simulink model "SFS0"  (R2022b)
settings: Solver=FixedStepAuto  StartTime=0.0  StopTime=10.0  FixedStep=0.20000000000000001  RelTol=1e-3
undefined symbols (not defined in the file): ACCELERATION_MAX, covA, covarience_matrix_IC, covG, covM, covP, covV, fusion_t, gps_ratio, location_lla_IC, MAG_MAX, noise_state, POS_MAX, state_IC, VELOCITY_MAX, YAW_MAX
settings Model: DVExtractedSubsystem=SFS  Creator=Inver  LastModifiedBy=Inver
settings DebuggingCC: SignalRangeChecking=warning  FrameProcessingCompatibilityMsg=none
settings RTWCC: TLCOptions=-aAlwaysIncludeCustomSrc=1

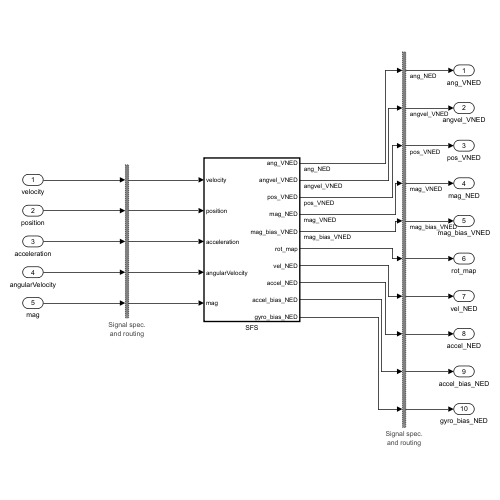
[thumbnail: Simulink's stored preview of the top-level diagram]
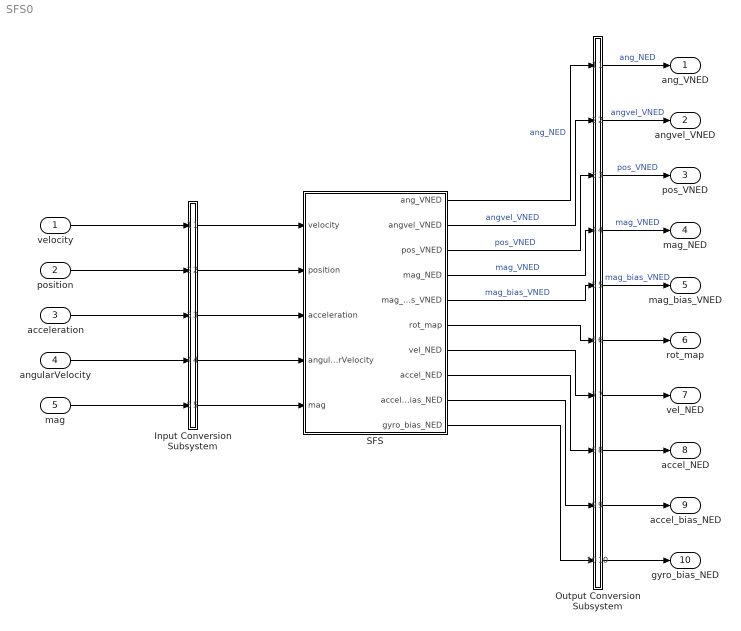
== system SFS0 ==
  velocity : Inport  OutMin=-30  OutMax=30  OutDataTypeStr=double  PortDimensions=[3, 1]  SampleTime=0.2  Interpolate=off
  position : Inport  Port=2  OutMin=-300  OutMax=300  OutDataTypeStr=double  PortDimensions=[3, 1]  SampleTime=0.2  Interpolate=off
  acceleration : Inport  Port=3  OutMin=-30  OutMax=30  OutDataTypeStr=double  PortDimensions=[3, 1]  SampleTime=0.2  Interpolate=off
  angularVelocity : Inport  Port=4  OutMin=-2.5  OutMax=2.5  OutDataTypeStr=double  PortDimensions=[3, 1]  SampleTime=0.2  Interpolate=off
  mag : Inport  Port=5  OutMin=-200  OutMax=200  OutDataTypeStr=double  PortDimensions=[3, 1]  SampleTime=0.2  Interpolate=off
  Input Conversion Subsystem : Subsystem  Tag=__SLT_ICS__  Description=|
      | Signal spec.
      | and routing
      settings: AttributesFormatString=%<Description>
  Output Conversion Subsystem : Subsystem  Tag=__SLT_OCS__  Description=|
      | Signal spec.
      | and routing
      settings: AttributesFormatString=%<Description>
  SFS : Subsystem  TreatAsAtomicUnit=on
  ang_VNED : Outport
  angvel_VNED : Outport  Port=2
  pos_VNED : Outport  Port=3
  mag_NED : Outport  Port=4
  mag_bias_VNED : Outport  Port=5
  rot_map : Outport  Port=6
  vel_NED : Outport  Port=7
  accel_NED : Outport  Port=8
  accel_bias_NED : Outport  Port=9
  gyro_bias_NED : Outport  Port=10
  wires:
  velocity/1 -> Input Conversion Subsystem/1(Inport_1)
  position/1 -> Input Conversion Subsystem/2(Inport_2)
  acceleration/1 -> Input Conversion Subsystem/3(Inport_3)
  angularVelocity/1 -> Input Conversion Subsystem/4(Inport_4)
  mag/1 -> Input Conversion Subsystem/5(Inport_5)
  Output Conversion Subsystem/1(Outport_1) -> ang_VNED/1  "ang_NED"
  Output Conversion Subsystem/2(Outport_2) -> angvel_VNED/1  "angvel_VNED"
  Output Conversion Subsystem/3(Outport_3) -> pos_VNED/1  "pos_VNED"
  Output Conversion Subsystem/4(Outport_4) -> mag_NED/1  "mag_VNED"
  Output Conversion Subsystem/5(Outport_5) -> mag_bias_VNED/1  "mag_bias_VNED"
  Output Conversion Subsystem/6(Outport_6) -> rot_map/1
  Output Conversion Subsystem/7(Outport_7) -> vel_NED/1
  Output Conversion Subsystem/8(Outport_8) -> accel_NED/1
  Output Conversion Subsystem/9(Outport_9) -> accel_bias_NED/1
  Output Conversion Subsystem/10(Outport_10) -> gyro_bias_NED/1
  Input Conversion Subsystem/1(Outport_1) -> SFS/1(velocity)
  Input Conversion Subsystem/2(Outport_2) -> SFS/2(position)
  Input Conversion Subsystem/3(Outport_3) -> SFS/3(acceleration)
  Input Conversion Subsystem/4(Outport_4) -> SFS/4(angularVelocity)
  Input Conversion Subsystem/5(Outport_5) -> SFS/5(mag)
  SFS/1(ang_VNED) -> Output Conversion Subsystem/1(Inport_1)  "ang_NED"
  SFS/2(angvel_VNED) -> Output Conversion Subsystem/2(Inport_2)  "angvel_VNED"
  SFS/3(pos_VNED) -> Output Conversion Subsystem/3(Inport_3)  "pos_VNED"
  SFS/4(mag_NED) -> Output Conversion Subsystem/4(Inport_4)  "mag_VNED"
  SFS/5(mag_bias_VNED) -> Output Conversion Subsystem/5(Inport_5)  "mag_bias_VNED"
  SFS/6(rot_map) -> Output Conversion Subsystem/6(Inport_6)
  SFS/7(vel_NED) -> Output Conversion Subsystem/7(Inport_7)
  SFS/8(accel_NED) -> Output Conversion Subsystem/8(Inport_8)
  SFS/9(accel_bias_NED) -> Output Conversion Subsystem/9(Inport_9)
  SFS/10(gyro_bias_NED) -> Output Conversion Subsystem/10(Inport_10)

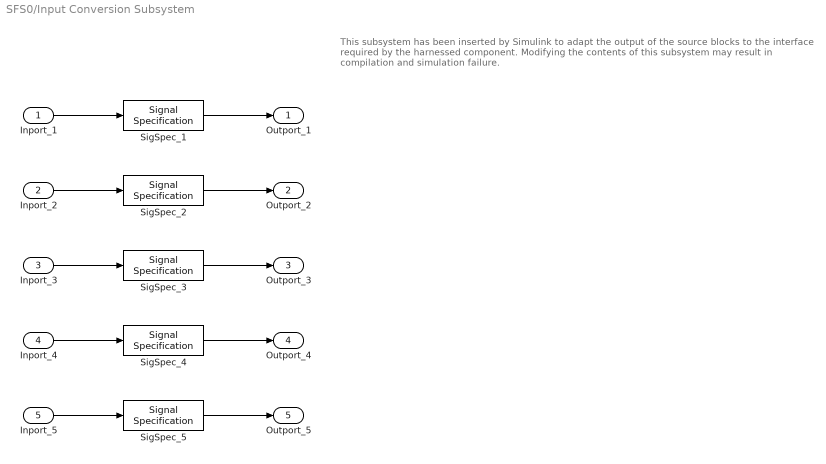
== system SFS0/Input Conversion Subsystem ==
  note: This subsystem has been inserted by Simulink to adapt the output of the source blocks to the interface required by the harnessed component.
      |  Modifying the contents of this subsystem may result in compilation and simulation failure.
  Inport_1 : Inport
  Inport_2 : Inport  Port=2
  Inport_3 : Inport  Port=3
  Inport_4 : Inport  Port=4
  Inport_5 : Inport  Port=5
  SigSpec_{1..5} (5 alike) : SignalSpecification  OutDataTypeStr=double  Dimensions=[3, 1]  SampleTime=0.2
  Outport_1 : Outport
  Outport_2 : Outport  Port=2
  Outport_3 : Outport  Port=3
  Outport_4 : Outport  Port=4
  Outport_5 : Outport  Port=5
  wires:
  SigSpec_1/1 -> Outport_1/1
  Inport_1/1 -> SigSpec_1/1
  SigSpec_2/1 -> Outport_2/1
  Inport_2/1 -> SigSpec_2/1
  SigSpec_3/1 -> Outport_3/1
  Inport_3/1 -> SigSpec_3/1
  SigSpec_4/1 -> Outport_4/1
  Inport_4/1 -> SigSpec_4/1
  SigSpec_5/1 -> Outport_5/1
  Inport_5/1 -> SigSpec_5/1

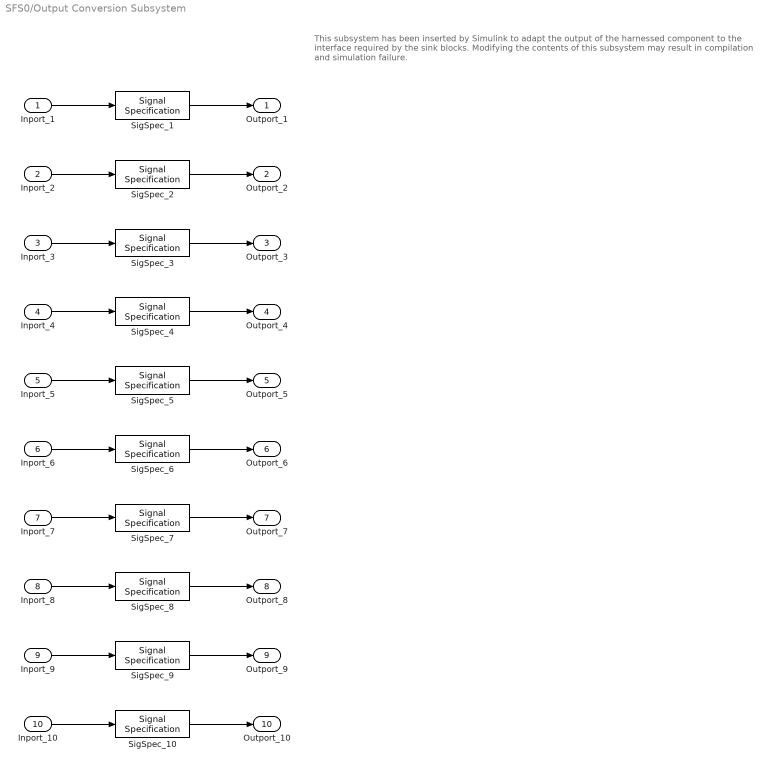
== system SFS0/Output Conversion Subsystem ==
  note: This subsystem has been inserted by Simulink to adapt the output of the harnessed component to the interface required by the sink blocks.
      |  Modifying the contents of this subsystem may result in compilation and simulation failure.
  Inport_1 : Inport
  Inport_2 : Inport  Port=2
  Inport_3 : Inport  Port=3
  Inport_4 : Inport  Port=4
  Inport_5 : Inport  Port=5
  Inport_6 : Inport  Port=6
  Inport_7 : Inport  Port=7
  Inport_8 : Inport  Port=8
  Inport_9 : Inport  Port=9
  Inport_10 : Inport  Port=10
  SigSpec_1 : SignalSpecification  OutDataTypeStr=double  Dimensions=[4, 1]  SampleTime=0.2
  SigSpec_{2..5,7..10} (8 alike) : SignalSpecification  OutDataTypeStr=double  Dimensions=[3, 1]  SampleTime=0.2
  SigSpec_6 : SignalSpecification  OutDataTypeStr=double  Dimensions=[3, 3]  SampleTime=0.2
  Outport_1 : Outport
  Outport_2 : Outport  Port=2
  Outport_3 : Outport  Port=3
  Outport_4 : Outport  Port=4
  Outport_5 : Outport  Port=5
  Outport_6 : Outport  Port=6
  Outport_7 : Outport  Port=7
  Outport_8 : Outport  Port=8
  Outport_9 : Outport  Port=9
  Outport_10 : Outport  Port=10
  wires:
  Inport_1/1 -> SigSpec_1/1
  SigSpec_1/1 -> Outport_1/1
  Inport_2/1 -> SigSpec_2/1
  SigSpec_2/1 -> Outport_2/1
  Inport_3/1 -> SigSpec_3/1
  SigSpec_3/1 -> Outport_3/1
  Inport_4/1 -> SigSpec_4/1
  SigSpec_4/1 -> Outport_4/1
  Inport_5/1 -> SigSpec_5/1
  SigSpec_5/1 -> Outport_5/1
  Inport_6/1 -> SigSpec_6/1
  SigSpec_6/1 -> Outport_6/1
  Inport_7/1 -> SigSpec_7/1
  SigSpec_7/1 -> Outport_7/1
  Inport_8/1 -> SigSpec_8/1
  SigSpec_8/1 -> Outport_8/1
  Inport_9/1 -> SigSpec_9/1
  SigSpec_9/1 -> Outport_9/1
  Inport_10/1 -> SigSpec_10/1
  SigSpec_10/1 -> Outport_10/1

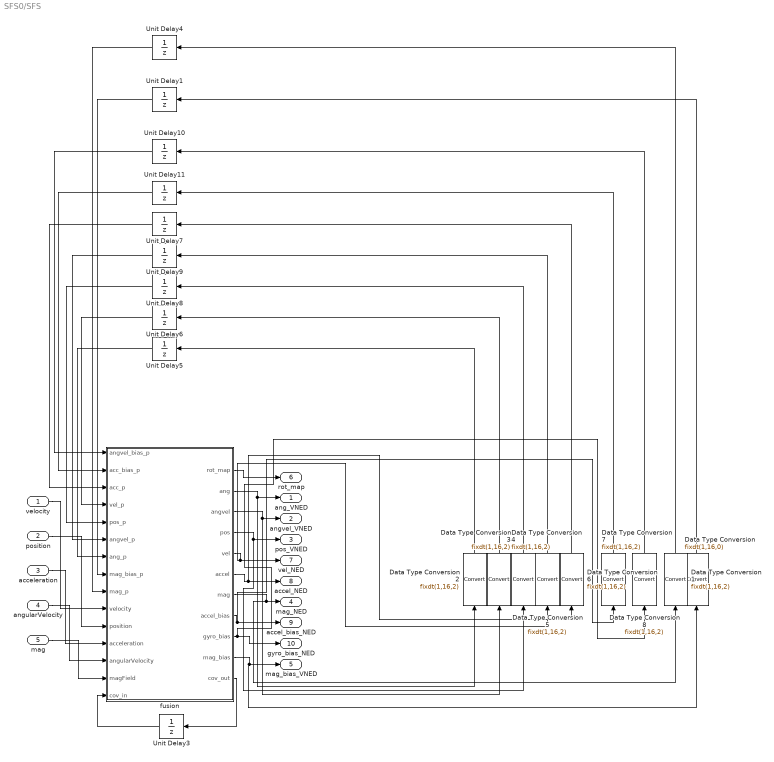
== system SFS0/SFS ==
  velocity : Inport  OutMin=-VELOCITY_MAX  OutMax=VELOCITY_MAX  OutDataTypeStr=double
  position : Inport  Port=2  OutMin=-POS_MAX  OutMax=POS_MAX  OutDataTypeStr=double
  acceleration : Inport  Port=3  OutMin=-ACCELERATION_MAX  OutMax=ACCELERATION_MAX  OutDataTypeStr=double  PortDimensions=[3 1]
  angularVelocity : Inport  Port=4  OutMin=-YAW_MAX  OutMax=YAW_MAX  OutDataTypeStr=double  PortDimensions=[3 1]
  mag : Inport  Port=5  OutMin=-MAG_MAX  OutMax=MAG_MAX  OutDataTypeStr=double  PortDimensions=[3 1]
  Data Type Conversion : DataTypeConversion  OutDataTypeStr=fixdt(1,16,0)  SaturateOnIntegerOverflow=off  RndMeth=Floor
  Data Type Conversion{1..8} (8 alike) : DataTypeConversion  OutDataTypeStr=fixdt(1,16,2)  SaturateOnIntegerOverflow=off  RndMeth=Floor
  Unit Delay1 : UnitDelay  InitialCondition=[0; 0; 0]  SampleTime=-1  HasFrameUpgradeWarning=on
  Unit Delay10 : UnitDelay  InitialCondition=state_IC(20:22)  SampleTime=-1  HasFrameUpgradeWarning=on
  Unit Delay11 : UnitDelay  InitialCondition=state_IC(17:19)  SampleTime=-1  HasFrameUpgradeWarning=on
  Unit Delay3 : UnitDelay  InitialCondition=covarience_matrix_IC  SampleTime=-1  HasFrameUpgradeWarning=on
  Unit Delay4 : UnitDelay  InitialCondition=mag_field_IC'  SampleTime=-1  HasFrameUpgradeWarning=on
  Unit Delay5 : UnitDelay  InitialCondition=state_IC(1:4)  SampleTime=-1  HasFrameUpgradeWarning=on
  Unit Delay6 : UnitDelay  InitialCondition=state_IC(5:7)  SampleTime=-1  HasFrameUpgradeWarning=on
  Unit Delay7 : UnitDelay  InitialCondition=state_IC(14:16)  SampleTime=-1  HasFrameUpgradeWarning=on
  Unit Delay8 : UnitDelay  InitialCondition=state_IC(8:10)  SampleTime=-1  HasFrameUpgradeWarning=on
  Unit Delay9 : UnitDelay  InitialCondition=state_IC(11:13)  SampleTime=-1  HasFrameUpgradeWarning=on
  fusion : MATLAB Function  TreatAsAtomicUnit=on
  ang_VNED : Outport  OutMin=-1  OutMax=1  OutDataTypeStr=double
  angvel_VNED : Outport  Port=2  OutMin=-YAW_MAX  OutMax=YAW_MAX  OutDataTypeStr=double
  pos_VNED : Outport  Port=3  OutMin=-POS_MAX  OutMax=POS_MAX  OutDataTypeStr=double
  mag_NED : Outport  Port=4  OutMin=-MAG_MAX  OutMax=MAG_MAX  OutDataTypeStr=double
  mag_bias_VNED : Outport  Port=5  OutMin=-MAG_MAX  OutMax=MAG_MAX  OutDataTypeStr=double
  rot_map : Outport  Port=6  OutMin=-1  OutMax=1  OutDataTypeStr=double
  vel_NED : Outport  Port=7  OutMin=-VELOCITY_MAX  OutMax=VELOCITY_MAX  OutDataTypeStr=double
  accel_NED : Outport  Port=8  OutMin=-ACCELERATION_MAX  OutMax=ACCELERATION_MAX  OutDataTypeStr=double
  accel_bias_NED : Outport  Port=9  OutMin=-ACCELERATION_MAX  OutMax=ACCELERATION_MAX  OutDataTypeStr=double
  gyro_bias_NED : Outport  Port=10  OutMin=-YAW_MAX  OutMax=YAW_MAX  OutDataTypeStr=double
  wires:
  Data Type Conversion8/1 -> Unit Delay10/1
  Data Type Conversion7/1 -> Unit Delay11/1
  Unit Delay10/1 -> fusion/1(angvel_bias_p)
  Unit Delay11/1 -> fusion/2(acc_bias_p)
  fusion/8(accel_bias) -> accel_bias_NED/1, Data Type Conversion7/1
  Unit Delay5/1 -> fusion/7(ang_p)
  Unit Delay9/1 -> fusion/6(angvel_p)
  Unit Delay8/1 -> fusion/5(pos_p)
  Unit Delay6/1 -> fusion/4(vel_p)
  Unit Delay7/1 -> fusion/3(acc_p)
  Data Type Conversion6/1 -> Unit Delay7/1
  Data Type Conversion5/1 -> Unit Delay9/1
  Data Type Conversion4/1 -> Unit Delay8/1
  Data Type Conversion3/1 -> Unit Delay6/1
  Data Type Conversion2/1 -> Unit Delay5/1
  Unit Delay1/1 -> fusion/8(mag_bias_p)
  Unit Delay4/1 -> fusion/9(mag_p)
  fusion/10(mag_bias) -> Data Type Conversion/1, mag_bias_VNED/1
  Data Type Conversion1/1 -> Unit Delay4/1
  Data Type Conversion/1 -> Unit Delay1/1
  fusion/9(gyro_bias) -> gyro_bias_NED/1, Data Type Conversion8/1
  fusion/7(mag) -> mag_NED/1, Data Type Conversion1/1
  fusion/6(accel) -> Data Type Conversion6/1, accel_NED/1
  fusion/5(vel) -> Data Type Conversion5/1, vel_NED/1
  fusion/4(pos) -> Data Type Conversion4/1, pos_VNED/1
  fusion/3(angvel) -> Data Type Conversion3/1, angvel_VNED/1
  fusion/2(ang) -> Data Type Conversion2/1, ang_VNED/1
  mag/1 -> fusion/14(magField)
  fusion/1(rot_map) -> rot_map/1
  velocity/1 -> fusion/10(velocity)
  acceleration/1 -> fusion/12(acceleration)
  position/1 -> fusion/11(position)
  Unit Delay3/1 -> fusion/15(cov_in)
  fusion/11(cov_out) -> Unit Delay3/1
  angularVelocity/1 -> fusion/13(angularVelocity)

== matlab function SFS0/SFS/fusion ==
  data: angvel_bias_p input; acc_bias_p input; acc_p input; vel_p input; pos_p input; angvel_p input; ang_p input; mag_bias_p input; mag_p input; rot_map output [-1..1]; ang output; angvel output; pos output; vel output; accel output; mag output; accel_bias output; gyro_bias output; mag_bias output; velocity input size=[3 1] [-VELOCITY_MAX..VELOCITY_MAX]; position input size=[3 1] [-POS_MAX..POS_MAX]; acceleration input size=[3 1] [-ACCELERATION_MAX..ACCELERATION_MAX]; angularVelocity input size=[3 1] [-YAW_MAX..YAW_MAX]; magField input size=[3 1] [-MAG_MAX..MAG_MAX]; cov_in input [-10..10]; covG parameter; covA parameter; covM parameter; covP parameter; covV parameter; fusion_t parameter; location_lla_IC parameter; cov_out output [-10..10]; noise_state parameter; gps_ratio parameter
function [rot_map, ang, angvel, pos, vel, accel, mag, accel_bias, gyro_bias, mag_bias, cov_out] = fusion(angvel_bias_p,acc_bias_p,acc_p, vel_p, pos_p, angvel_p, ang_p, mag_bias_p, mag_p, velocity, position ,acceleration,angularVelocity, magField, cov_in, covG, covA, covM, covP, covV, fusion_t, location_lla_IC, noise_state, gps_ratio) 
%% Create Filter
filter = insfilterAsync();
filter.ReferenceLocation = location_lla_IC;
%filter.State(1:22) = state_in;
filter.StateCovariance = cov_in;

filter.State(1:4) = ang_p;
filter.State(5:7) = angvel_p;
filter.State(8:10) = pos_p;
filter.State(11:13) = vel_p;
filter.State(14:16) = acc_p;
filter.State(17:19) = acc_bias_p;
filter.State(20:22) = angvel_bias_p;
filter.State(23:25) = mag_p;
filter.State(26:28) = mag_bias_p;

filter.QuaternionNoise = noise_state(1:4);
filter.AngularVelocityNoise = noise_state(5:7);
filter.PositionNoise = noise_state(8:10);
filter.VelocityNoise = noise_state(11:13);
filter.AccelerationNoise = noise_state(14:16);
filter.GyroscopeBiasNoise = noise_state(17:19);
filter.AccelerometerBiasNoise = noise_state(20:22);
filter.GeomagneticVectorNoise = noise_state(23:25);
filter.MagnetometerBiasNoise = noise_state(26:28);

%% Sensor Fusion
predict(filter, fusion_t);

fuseaccel(filter,acceleration',covA);
fusegyro(filter,angularVelocity',covG);
fusemag(filter, magField',covM);
fusegps(filter,position',covP,velocity',covV);

[~,rot_map,~] = pose(filter, 'rotmat');

%% Extract Individual Signals
% states
% state_out = filter.State;
cov_out = filter.StateCovariance;

% Vehicle POSE
ang = filter.State(1:4);                    % quaternion (VNED2SNED)
angvel = filter.State(5:7);                 % chassis angular velocity (rad/s)(VNED)
pos = filter.State(8:10);                   % chassis position (m)(NED)
vel = filter.State(11:13);                  % chassis velocity (m/s)(VNED)
accel = filter.State(14:16);                % chassis acceleration (m/s^2)(VNED)
mag = filter.State(23:25);                  % magnetic field (uT)(NED)

% Sensor Parameters
accel_bias = filter.State(17:19);           % accelerometer bias (m/s^2)(VNED)
gyro_bias = filter.State(20:22);            % gyroscope bias (rad/s)(VNED)
mag_bias = filter.State(26:28);             % magnetometer bias (uT)(NED)

end
